simulink model "ask(1)"  (R2014a)
settings: Solver=ode45  StartTime=0.0  StopTime=10.0  RelTol=1e-3
settings Model: Creator=mm  LastModifiedBy=mm

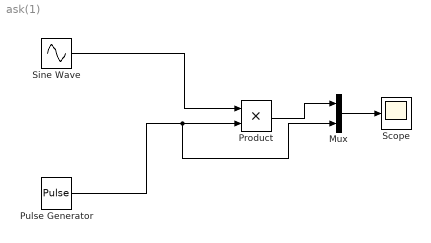
== system ask(1) ==
  Mux : Mux  Inputs=2
  Product : Product
  Pulse Generator : DiscretePulseGenerator  PulseType=Time based  PulseWidth=50
  Scope : Scope
  Sine Wave : Sin  Frequency=100  SampleTime=0.0001
  wires:
  Pulse Generator/1 -> Mux/2, Product/2
  Sine Wave/1 -> Product/1
  Product/1 -> Mux/1
  Mux/1 -> Scope/1
